simulink model "ep4_1"  (R2023b)
settings: Solver=VariableStepAuto  StartTime=0.0  StopTime=50  MaxStep=0.01  RelTol=1e-3
settings Model: Creator=86186  LastModifiedBy=86186

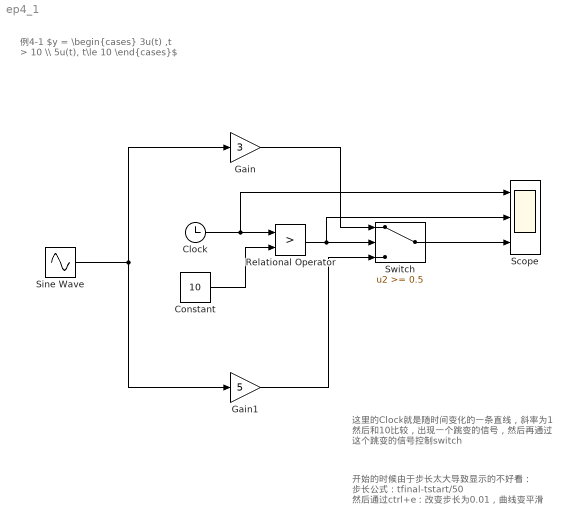
== system ep4_1 ==
  note: 开始的时候由于步长太大导致显示的不好看：
      | 步长公式：tfinal-tstart/50
      | 然后通过ctrl+e：改变步长为0.01，曲线变平滑
  note: 这里的Clock就是随时间变化的一条直线，斜率为1
      | 然后和10比较，出现一个跳变的信号，然后再通过
      | 这个跳变的信号控制switch
  note: 例4-1
      | $y = \begin{cases} 3u(t) ,t > 10 \\ 5u(t), t\le 10 \end{cases}$
  Clock : Clock
  Constant : Constant  Value=10
  Gain : Gain  Gain=3
  Gain1 : Gain  Gain=5
  Relational Operator : RelationalOperator  Operator=>  OutDataTypeStr=boolean  RndMeth=Simplest  InputSameDT=off
  Scope : Scope  NumInputPorts=3
  Sine Wave : Sin  SampleTime=0
  Switch : Switch  Threshold=0.5  SaturateOnIntegerOverflow=off  InputSameDT=off
  wires:
  Sine Wave/1 -> Gain/1, Gain1/1
  Gain/1 -> Switch/1
  Gain1/1 -> Switch/3
  Constant/1 -> Relational Operator/2
  Relational Operator/1 -> Scope/2, Switch/2
  Clock/1 -> Scope/1, Relational Operator/1
  Switch/1 -> Scope/3
